simulink model "p5"  (R2021b)
settings: Solver=VariableStepAuto  StartTime=0.0  StopTime=30  RelTol=1e-3
settings Model: Creator=hp  LastModifiedBy=hp

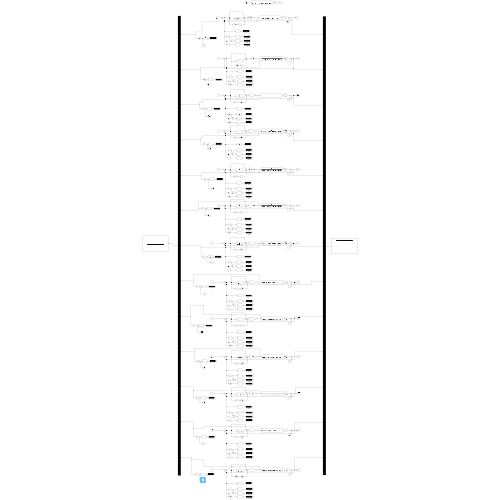
[thumbnail: Simulink's stored preview of the top-level diagram]
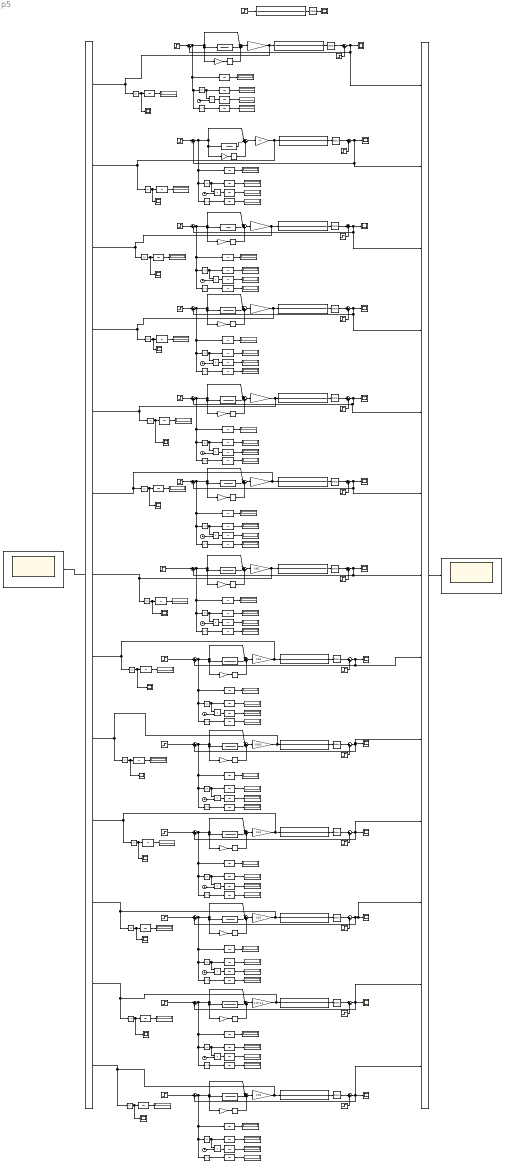
== system p5 ==
  {1..13} (13 alike) : Display
  Abs{,1..25} (26 alike) : Abs
  Clock{,1..12} (13 alike) : Clock
  Derivative{,1..12} (13 alike) : Derivative
  Divide{,1..12} (13 alike) : Product  Inputs=**
  Gain : Gain  Gain=1.2 / (2*0.8/1.4)
  Gain1 : Gain  Gain=0.5*0.8
  Gain10 : Gain  Gain=1.2*1.4 / (2*0.8)
  Gain11 : Gain  Gain=0.42*0.8
  Gain12 : Gain  Gain=0.8/2
  Gain13 : Gain  Gain=0.43*2.2
  Gain{14,18,20,24} (4 alike) : Gain  Gain=1.3/2
  Gain15 : Gain  Gain=0.43*2.2
  Gain16 : Gain  Gain=0.85/2
  Gain17 : Gain  Gain=0.06*2.2
  Gain19 : Gain  Gain=0.025*2.2
  Gain2 : Gain  Gain=1.05*((4/3) + 0.8/(4*1.05))/(2*0.8)
  Gain21 : Gain  Gain=2.6/8
  Gain22 : Gain  Gain=1.11*1.1
  Gain23 : Gain  Gain=3.11/9
  Gain25 : Gain  Gain=0.9*0.3
  Gain3 : Gain  Gain=0.8*4/(11+2*0.8/1.05)
  Gain4 : Gain  Gain=0.6*1.4 / (2*0.8)
  Gain5 : Gain  Gain=0.5*0.8
  Gain6 : Gain  Gain=0.95*1.4 / (2*0.8)
  Gain7 : Gain  Gain=0.47*0.8
  Gain8 : Gain  Gain=0.95*1.4 / (2*0.8)
  Gain9 : Gain  Gain=0.42*0.8
  IAE{1..13} (13 alike) : Display
  IE{1..13} (13 alike) : Display
  ISE{1..13} (13 alike) : Display
  ITAE{1..13} (13 alike) : Display
  Mux : Mux  Inputs=13
  Mux1 : Mux  Inputs=13
  Power{,1..12} (13 alike) : Math  Operator=square  SaturateOnIntegerOverflow=on
  Scope{,1..28} (29 alike) : Scope
  Step{,2,4..5,8,10,12,14,16,18,20,22,24,26} (14 alike) : Step  Time=0  SampleTime=0
  Step{1,3,6..7,9,11,13,15,17,19,21,23,25} (13 alike) : Step  Time=15  After=0.5  SampleTime=0
  Sum{,3,6,9,14,17,20,23,26,29,32,35,38} (13 alike) : Sum  Inputs=|++
  Sum{1,4,7,10,12,15,18,21,24,27,30,33,36} (13 alike) : Sum  Inputs=|+++
  Sum{2,5,8,11,13,16,19,22,25,28,31,34,37} (13 alike) : Sum  Inputs=|+-
  Transfer Fcn{,2,4,13,19,25,31,37,43,49,55,61,67,73} (14 alike) : TransferFcn  Numerator=[2]  Denominator=[0.000064 0.009984 0.25792 1.248 1]
  Transfer Fcn1 : TransferFcn  Denominator=[2*0.8 0]
  Transfer Fcn{5..12,15..18,21..24,27..30,33..36,39..42,45..48,51..54,57..60,63..66,69..72,75..91} (65 alike) : TransferFcn  Denominator=[1 0]
  Transfer Fcn14 : TransferFcn  Denominator=[1.4 0]
  Transfer Fcn20 : TransferFcn  Denominator=[1.4*1.4 0]
  Transfer Fcn26 : TransferFcn  Denominator=[2.4*0.8 0]
  Transfer Fcn3 : TransferFcn  Denominator=[0.8*(32+6*0.8/1.05)/(13+8*0.8/1.05) 0]
  Transfer Fcn32 : TransferFcn  Denominator=[2*0.8 0]
  Transfer Fcn38 : TransferFcn  Denominator=[0.48*2.2 0]
  Transfer Fcn44 : TransferFcn  Denominator=[0.48*2.2 0]
  Transfer Fcn50 : TransferFcn  Denominator=[0.8*2.2 0]
  Transfer Fcn56 : TransferFcn  Denominator=[0.7*2.2 0]
  Transfer Fcn62 : TransferFcn  Denominator=[2.6/2 0]
  Transfer Fcn68 : TransferFcn  Denominator=[3.11/3.6 0]
  Transfer Fcn74 : TransferFcn  Denominator=[0.7*3.3 0]
  Transport Delay{,1..13} (14 alike) : TransportDelay  DelayTime=0.633
  wires:
  Transfer Fcn/1 -> Transport Delay/1
  Gain/1 -> Abs13/1, Mux1/1, Transfer Fcn/1
  Transport Delay/1 -> Sum/1
  Step1/1 -> Sum/2
  Transfer Fcn1/1 -> Sum1/2
  Derivative/1 -> Sum1/3
  Gain1/1 -> Derivative/1
  Sum1/1 -> Gain/1
  Step/1 -> Sum2/1
  Sum2/1 -> Power/1, Abs/1, Transfer Fcn5/1, Sum1/1, Gain1/1, Transfer Fcn1/1
  Derivative1/1 -> Sum4/3
  Step3/1 -> Sum3/2
  Transfer Fcn3/1 -> Sum4/2
  Gain3/1 -> Derivative1/1
  Step2/1 -> Sum5/1
  Sum3/1 -> Mux/2, Sum5/2, Scope1/1  "CC"
  Transfer Fcn2/1 -> Transport Delay1/1
  Transport Delay1/1 -> Sum3/1
  Sum4/1 -> Gain2/1
  Transfer Fcn4/1 -> Transport Delay2/1
  Step4/1 -> Transfer Fcn4/1
  Transport Delay2/1 -> Scope/1
  Sum/1 -> Mux/1, Sum2/2, Scope2/1  "ZN_Open"
  Abs/1 -> Divide/1, Transfer Fcn6/1
  Power/1 -> Transfer Fcn7/1
  Clock/1 -> Divide/2
  Divide/1 -> Transfer Fcn8/1
  Transfer Fcn5/1 -> IE1/1  "IE"
  Transfer Fcn6/1 -> IAE1/1  "IAE"
  Transfer Fcn8/1 -> ITAE1/1  "ITAE"
  Transfer Fcn7/1 -> ISE1/1  "ISE"
  Transfer Fcn12/1 -> ITAE2/1  "ITAE"
  Sum5/1 -> Sum4/1, Gain3/1, Transfer Fcn3/1, Transfer Fcn9/1, Power1/1, Abs1/1
  Abs1/1 -> Divide1/1, Transfer Fcn10/1
  Divide1/1 -> Transfer Fcn12/1
  Transfer Fcn10/1 -> IAE2/1  "IAE"
  Clock1/1 -> Divide1/2
  Transfer Fcn9/1 -> IE2/1  "IE"
  Transfer Fcn11/1 -> ISE2/1  "ISE"
  Power1/1 -> Transfer Fcn11/1
  Derivative2/1 -> Sum7/3
  Step6/1 -> Sum6/2
  Transfer Fcn14/1 -> Sum7/2
  Step5/1 -> Sum8/1
  Transfer Fcn18/1 -> ITAE3/1  "ITAE"
  Gain5/1 -> Derivative2/1
  Sum6/1 -> Scope3/1, Mux/3, Sum8/2  "CHR_r0"
  Sum8/1 -> Power2/1, Abs2/1, Transfer Fcn15/1, Sum7/1, Gain5/1, Transfer Fcn14/1
  Abs2/1 -> Divide2/1, Transfer Fcn16/1
  Transfer Fcn17/1 -> ISE3/1  "ISE"
  Power2/1 -> Transfer Fcn17/1
  Divide2/1 -> Transfer Fcn18/1
  Clock2/1 -> Divide2/2
  Transfer Fcn15/1 -> IE3/1  "IE"
  Transfer Fcn13/1 -> Transport Delay3/1
  Transport Delay3/1 -> Sum6/1
  Sum7/1 -> Gain4/1
  Transfer Fcn16/1 -> IAE3/1  "IAE"
  Power3/1 -> Transfer Fcn23/1
  Transport Delay4/1 -> Sum9/1
  Transfer Fcn21/1 -> IE4/1  "IE"
  Abs3/1 -> Divide3/1, Transfer Fcn22/1
  Divide3/1 -> Transfer Fcn24/1
  Transfer Fcn23/1 -> ISE4/1  "ISE"
  Clock3/1 -> Divide3/2
  Sum11/1 -> Power3/1, Abs3/1, Transfer Fcn21/1, Sum10/1, Gain7/1, Transfer Fcn20/1
  Transfer Fcn22/1 -> IAE4/1  "IAE"
  Gain7/1 -> Derivative3/1
  Transfer Fcn24/1 -> ITAE4/1  "ITAE"
  Sum10/1 -> Gain6/1
  Sum9/1 -> Scope4/1, Mux/4, Sum11/2  "CHR_r20"
  Derivative3/1 -> Sum10/3
  Transfer Fcn19/1 -> Transport Delay4/1
  Transfer Fcn20/1 -> Sum10/2
  Step7/1 -> Sum9/2
  Step8/1 -> Sum11/1
  Step9/1 -> Sum14/2
  Transfer Fcn25/1 -> Transport Delay5/1
  Derivative4/1 -> Sum12/3
  Sum14/1 -> Scope5/1, Mux/5, Sum13/2  "CHR_d0"
  Sum12/1 -> Gain8/1
  Transfer Fcn26/1 -> Sum12/2
  Transfer Fcn30/1 -> ITAE5/1  "ITAE"
  Transfer Fcn28/1 -> IAE5/1  "IAE"
  Sum13/1 -> Power4/1, Abs4/1, Transfer Fcn27/1, Sum12/1, Gain9/1, Transfer Fcn26/1
  Gain9/1 -> Derivative4/1
  Clock4/1 -> Divide4/2
  Transfer Fcn29/1 -> ISE5/1  "ISE"
  Divide4/1 -> Transfer Fcn30/1
  Abs4/1 -> Divide4/1, Transfer Fcn28/1
  Transfer Fcn27/1 -> IE5/1  "IE"
  Transport Delay5/1 -> Sum14/1
  Step10/1 -> Sum13/1
  Power4/1 -> Transfer Fcn29/1
  Step11/1 -> Sum17/2
  Transfer Fcn31/1 -> Transport Delay6/1
  Derivative5/1 -> Sum15/3
  Sum17/1 -> Scope6/1, Mux/6, Sum16/2  "CHR_d20"
  Sum15/1 -> Gain10/1
  Transfer Fcn32/1 -> Sum15/2
  Transfer Fcn36/1 -> ITAE6/1  "ITAE"
  Transfer Fcn34/1 -> IAE6/1  "IAE"
  Sum16/1 -> Power5/1, Abs5/1, Transfer Fcn33/1, Sum15/1, Gain11/1, Transfer Fcn32/1
  Gain11/1 -> Derivative5/1
  Clock5/1 -> Divide5/2
  Transfer Fcn35/1 -> ISE6/1  "ISE"
  Divide5/1 -> Transfer Fcn36/1
  Abs5/1 -> Divide5/1, Transfer Fcn34/1
  Transfer Fcn33/1 -> IE6/1  "IE"
  Transport Delay6/1 -> Sum17/1
  Step12/1 -> Sum16/1
  Power5/1 -> Transfer Fcn35/1
  Step14/1 -> Sum19/1
  Power6/1 -> Transfer Fcn41/1
  Gain13/1 -> Derivative6/1
  Transfer Fcn41/1 -> ISE7/1  "ISE"
  Abs6/1 -> Divide6/1, Transfer Fcn40/1
  Transfer Fcn39/1 -> IE7/1  "IE"
  Sum18/1 -> Gain12/1
  Clock6/1 -> Divide6/2
  Divide6/1 -> Transfer Fcn42/1
  Transfer Fcn40/1 -> IAE7/1  "IAE"
  Step13/1 -> Sum20/2
  Sum19/1 -> Power6/1, Abs6/1, Transfer Fcn39/1, Sum18/1, Gain13/1, Transfer Fcn38/1
  Transfer Fcn42/1 -> ITAE7/1  "ITAE"
  Sum20/1 -> Scope7/1, Mux/7, Sum19/2  "fertik_r"
  Transport Delay7/1 -> Sum20/1
  Derivative6/1 -> Sum18/3
  Transfer Fcn37/1 -> Transport Delay7/1
  Transfer Fcn38/1 -> Sum18/2
  Transfer Fcn44/1 -> Sum21/2
  Transport Delay8/1 -> Sum23/1
  Derivative7/1 -> Sum21/3
  Transfer Fcn48/1 -> ITAE8/1  "ITAE"
  Sum23/1 -> Scope8/1, Mux/8, Sum22/2  "fertik_d"
  Sum21/1 -> Gain14/1
  Transfer Fcn46/1 -> IAE8/1  "IAE"
  Clock7/1 -> Divide7/2
  Divide7/1 -> Transfer Fcn48/1
  Transfer Fcn45/1 -> IE8/1  "IE"
  Transfer Fcn47/1 -> ISE8/1  "ISE"
  Transfer Fcn43/1 -> Transport Delay8/1
  Gain15/1 -> Derivative7/1
  Step15/1 -> Sum23/2
  Power7/1 -> Transfer Fcn47/1
  Sum22/1 -> Power7/1, Abs7/1, Transfer Fcn45/1, Sum21/1, Gain15/1, Transfer Fcn44/1
  Step16/1 -> Sum22/1
  Abs7/1 -> Divide7/1, Transfer Fcn46/1
  Transfer Fcn50/1 -> Sum24/2
  Transport Delay9/1 -> Sum26/1
  Derivative8/1 -> Sum24/3
  Transfer Fcn54/1 -> ITAE9/1  "ITAE"
  Sum26/1 -> Mux/9, Scope9/1, Sum25/2  "Ciancone Marline_r"
  Sum24/1 -> Gain16/1
  Transfer Fcn52/1 -> IAE9/1  "IAE"
  Clock8/1 -> Divide8/2
  Divide8/1 -> Transfer Fcn54/1
  Transfer Fcn51/1 -> IE9/1  "IE"
  Transfer Fcn53/1 -> ISE9/1  "ISE"
  Transfer Fcn49/1 -> Transport Delay9/1
  Gain17/1 -> Derivative8/1
  Step17/1 -> Sum26/2
  Power8/1 -> Transfer Fcn53/1
  Sum25/1 -> Power8/1, Abs8/1, Transfer Fcn51/1, Sum24/1, Gain17/1, Transfer Fcn50/1
  Step18/1 -> Sum25/1
  Abs8/1 -> Divide8/1, Transfer Fcn52/1
  Abs9/1 -> Divide9/1, Transfer Fcn58/1
  Step20/1 -> Sum28/1
  Sum28/1 -> Power9/1, Abs9/1, Transfer Fcn57/1, Sum27/1, Gain19/1, Transfer Fcn56/1
  Power9/1 -> Transfer Fcn59/1
  Step19/1 -> Sum29/2
  Clock9/1 -> Divide9/2
  Transfer Fcn59/1 -> ISE10/1  "ISE"
  Gain19/1 -> Derivative9/1
  Transfer Fcn55/1 -> Transport Delay10/1
  Transfer Fcn57/1 -> IE10/1  "IE"
  Divide9/1 -> Transfer Fcn60/1
  Transfer Fcn60/1 -> ITAE10/1  "ITAE"
  Sum27/1 -> Gain18/1
  Derivative9/1 -> Sum27/3
  Sum29/1 -> Mux/10, Scope10/1, Sum28/2  "Ciancone Marline_d"
  Transport Delay10/1 -> Sum29/1
  Transfer Fcn56/1 -> Sum27/2
  Transfer Fcn58/1 -> IAE10/1  "IAE"
  Transfer Fcn64/1 -> IAE11/1  "IAE"
  Transport Delay11/1 -> Sum32/1
  Divide10/1 -> Transfer Fcn66/1
  Transfer Fcn66/1 -> ITAE11/1  "ITAE"
  Derivative10/1 -> Sum30/3
  Sum32/1 -> Mux/11, Scope11/1, Sum31/2  "ZN_closed"
  Transfer Fcn63/1 -> IE11/1  "IE"
  Gain21/1 -> Derivative10/1
  Clock10/1 -> Divide10/2
  Step21/1 -> Sum32/2
  Transfer Fcn65/1 -> ISE11/1  "ISE"
  Transfer Fcn61/1 -> Transport Delay11/1
  Transfer Fcn62/1 -> Sum30/2
  Sum31/1 -> Power10/1, Abs10/1, Transfer Fcn63/1, Gain21/1, Transfer Fcn62/1, Sum30/1
  Sum30/1 -> Gain20/1
  Abs10/1 -> Divide10/1, Transfer Fcn64/1
  Step22/1 -> Sum31/1
  Power10/1 -> Transfer Fcn65/1
  Step24/1 -> Sum34/1
  Abs11/1 -> Divide11/1, Transfer Fcn70/1
  Sum34/1 -> Power11/1, Abs11/1, Transfer Fcn69/1, Gain23/1, Transfer Fcn68/1, Sum33/1
  Step23/1 -> Sum35/2
  Transfer Fcn71/1 -> ISE12/1  "ISE"
  Transfer Fcn68/1 -> Sum33/2
  Transfer Fcn67/1 -> Transport Delay12/1
  Clock11/1 -> Divide11/2
  Gain23/1 -> Derivative11/1
  Divide11/1 -> Transfer Fcn72/1
  Sum35/1 -> Mux/12, Scope12/1, Sum34/2  "Damped Oscillation"
  Sum33/1 -> Gain22/1
  Transfer Fcn72/1 -> ITAE12/1  "ITAE"
  Transport Delay12/1 -> Sum35/1
  Power11/1 -> Transfer Fcn71/1
  Derivative11/1 -> Sum33/3
  Transfer Fcn70/1 -> IAE12/1  "IAE"
  Transfer Fcn69/1 -> IE12/1  "IE"
  Power12/1 -> Transfer Fcn77/1
  Derivative12/1 -> Sum36/3
  Sum36/1 -> Gain24/1
  Clock12/1 -> Divide12/2
  Transport Delay13/1 -> Sum38/1
  Divide12/1 -> Transfer Fcn78/1
  Transfer Fcn73/1 -> Transport Delay13/1
  Gain25/1 -> Derivative12/1
  Transfer Fcn77/1 -> ISE13/1  "ISE"
  Step25/1 -> Sum38/2
  Transfer Fcn78/1 -> ITAE13/1  "ITAE"
  Sum37/1 -> Power12/1, Abs12/1, Transfer Fcn75/1, Gain25/1, Transfer Fcn74/1, Sum36/1
  Transfer Fcn74/1 -> Sum36/2
  Step26/1 -> Sum37/1
  Sum38/1 -> Sum37/2, Mux/13, Scope13/1  "Process Respond"
  Transfer Fcn75/1 -> IE13/1  "IE"
  Abs12/1 -> Divide12/1, Transfer Fcn76/1
  Transfer Fcn76/1 -> IAE13/1  "IAE"
  Mux/1 -> Scope14/1
  Mux1/1 -> Scope15/1
  Abs13/1 -> Scope16/1, Transfer Fcn79/1
  Transfer Fcn79/1 -> 1/1  "IE"
  Transfer Fcn80/1 -> 2/1  "IE"
  Abs14/1 -> Scope17/1, Transfer Fcn80/1
  Gain2/1 -> Abs14/1, Mux1/2, Transfer Fcn2/1
  Transfer Fcn81/1 -> 3/1  "IE"
  Abs15/1 -> Scope18/1, Transfer Fcn81/1
  Gain4/1 -> Mux1/3, Abs15/1, Transfer Fcn13/1
  Transfer Fcn82/1 -> 4/1  "IE"
  Abs16/1 -> Scope19/1, Transfer Fcn82/1
  Gain6/1 -> Abs16/1, Mux1/4, Transfer Fcn19/1
  Transfer Fcn83/1 -> 5/1  "IE"
  Abs17/1 -> Scope20/1, Transfer Fcn83/1
  Gain8/1 -> Abs17/1, Mux1/5, Transfer Fcn25/1
  Transfer Fcn84/1 -> 6/1  "IE"
  Abs18/1 -> Scope21/1, Transfer Fcn84/1
  Gain10/1 -> Abs18/1, Mux1/6, Transfer Fcn31/1
  Transfer Fcn85/1 -> 7/1  "IE"
  Abs19/1 -> Scope22/1, Transfer Fcn85/1
  Gain12/1 -> Abs19/1, Mux1/7, Transfer Fcn37/1
  Transfer Fcn86/1 -> 8/1  "IE"
  Abs20/1 -> Scope23/1, Transfer Fcn86/1
  Gain14/1 -> Abs20/1, Mux1/8, Transfer Fcn43/1
  Transfer Fcn87/1 -> 9/1  "IE"
  Abs21/1 -> Scope24/1, Transfer Fcn87/1
  Gain16/1 -> Abs21/1, Mux1/9, Transfer Fcn49/1
  Transfer Fcn88/1 -> 10/1  "IE"
  Abs22/1 -> Scope25/1, Transfer Fcn88/1
  Gain18/1 -> Abs22/1, Mux1/10, Transfer Fcn55/1
  Transfer Fcn89/1 -> 13/1  "IE"
  Abs23/1 -> Scope28/1, Transfer Fcn89/1
  Gain24/1 -> Abs23/1, Mux1/13, Transfer Fcn73/1
  Transfer Fcn90/1 -> 12/1  "IE"
  Abs24/1 -> Scope27/1, Transfer Fcn90/1
  Gain22/1 -> Abs24/1, Mux1/12, Transfer Fcn67/1
  Transfer Fcn91/1 -> 11/1  "IE"
  Abs25/1 -> Scope26/1, Transfer Fcn91/1
  Gain20/1 -> Abs25/1, Mux1/11, Transfer Fcn61/1
